simulink model "EvitarObstaculo"  (R2023a)
settings: Solver=FixedStepAuto  StartTime=0.0  StopTime=100  FixedStep=Ts  RelTol=1e-3
values from neighbouring files (symbols this model uses):
  obsx = 3    [RunTrayectorias.m]
  obsy = 2    [RunTrayectorias.m]
  Ts = 100e-3    (= 0.1)    [RunTrayectorias.m]
undefined symbols (not defined in the file or in its folder): DiscIntNeverNeededParam, refx, refy
libraries: fuzblock x1
settings Model: Creator=Edu  LastModifiedBy=Edu
settings DataIOCC: ReturnWorkspaceOutputs=off

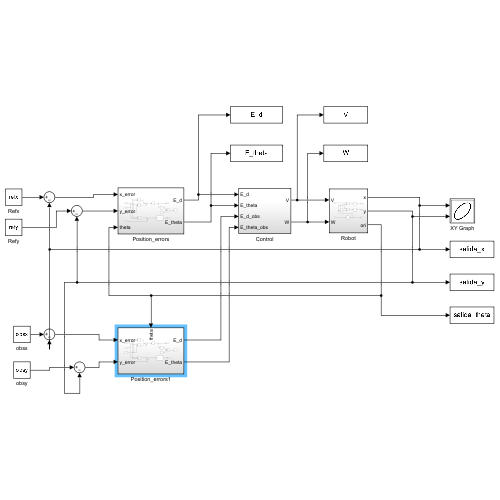
[thumbnail: Simulink's stored preview of the top-level diagram]
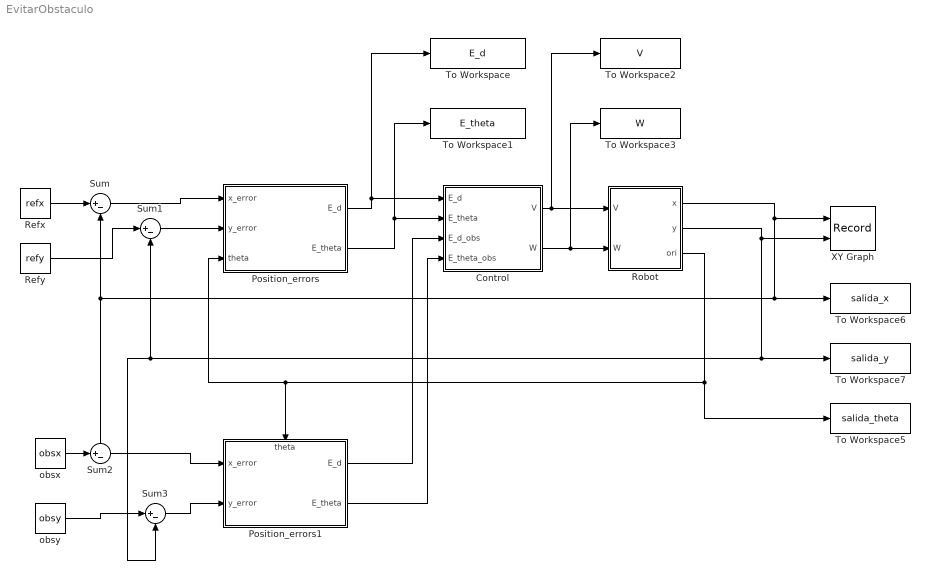
== system EvitarObstaculo ==
  Control : Subsystem
  Position_errors : Subsystem
  Position_errors1 : Subsystem
      settings: PortSchema="{\"entries\":[{\"content\":{\"sides\":[{\"content\":{\"connectorIds\":[\"In1\",\"In2\"]},\"type\":\"ConnectorPlacement.EquallySpacedRectSide\",\"uuid\":\"724a1adf-34fd-47e8-8329-3234fcffba95\"},{\"content\":{\"connectorIds\":[\"Out1\",\"Out2\"],\"side\":\"RIGHT\"},\"type\":\"ConnectorPlacement.EquallySpacedRectSide\",\"uuid\":\"8963bb18-06e6-4569-9caa-12a8dca62f16\"},{\"content\":{\"connectorIds\":[\"In3\"],\"side\":\"TOP\"},\"type\":\"ConnectorPlacement.EquallySpacedRectSide\",\"uuid\":\"b639e4b5-9e5a-472e-9105-86d06ea8a990\"}]},\"type\":\"ConnectorPlacement.EquallySpacedConnector\",\"uuid\":\"88dc6a9c-ca86-465e-ac65-937620f59bbe\"}],\"packageUris\":[\"http://schema.mathworks.com/mf0/Connector/R2020b\"],\"version\":\"1.0\"}"
  Refx : Constant  Value=refx
  Refy : Constant  Value=refy
  Robot : Subsystem
  Sum{,1..3} (4 alike) : Sum  Inputs=|+-
  To Workspace : ToWorkspace  VariableName=E_d  SaveFormat=Structure With Time  SampleTime=-1
  To Workspace1 : ToWorkspace  VariableName=E_theta  SaveFormat=Structure With Time  SampleTime=-1
  To Workspace2 : ToWorkspace  VariableName=V  SaveFormat=Structure With Time  SampleTime=-1
  To Workspace3 : ToWorkspace  VariableName=W  SaveFormat=Structure With Time  SampleTime=-1
  To Workspace5 : ToWorkspace  VariableName=salida_theta  SaveFormat=Structure With Time  SampleTime=-1
  To Workspace6 : ToWorkspace  VariableName=salida_x  SaveFormat=Structure With Time  SampleTime=-1
  To Workspace7 : ToWorkspace  VariableName=salida_y  SaveFormat=Structure With Time  SampleTime=-1
  XY Graph : Record  FileSettingsInternal="{\"entries\":[{\"content\":{\"excelSettings\":{\"content\":{},\"type\":\"Streamout.ExcelSettings\"}},\"type\":\"Streamout.FileSettingStorage\",\"uuid\":\"\"}],\"packageUris\":[\"http:\\/\\/schema.mathworks.com\\/mf0\\/streamout_blocks\\/R2020a\"],\"version\":\"1.0\"}"  Layout=[1 1]  SignalsInternal="{\"entries\":[{\"content\":{\"signals\":[{\"content\":{\"blockPath\":[],\"dimensions\":[1],\"domain\":\"\",\"lineColor\":\"#a2142f\",\"plots\":[1],\"port\":1,\"sid\":[\"\"],\"signalID\":3541,\"signalName\":\"Robot:1\"},\"type\":\"RecordBlkView.Signal\",\"uuid\":\"\"},{\"content\":{\"blockPath\":[],\"dimensions\":[1],\"domain\":\"\",\"lineColor\":\"#139fff\",\"plots\":[1],\"port\":2,\"sid\":[\"\"],\"signalID\":3545,\"signalName\":\"Robot:2\"},\"type\":\"RecordBlkView.Signal\",\"uuid\":\"\"}]},\"type\":\"RecordBlkView.InputSignals\",\"uuid\":\"\"}],\"packageUris\":[\"http:\\/\\/schema.mathworks.com\\/mf0\\/streamout_blocks\\/R2020a\"],\"version\":\"1.0\"}"  VisualizationBindings="{\"xyplotplugin\":{\"info\":[{\"series\":[{\"bindingParametersList\":[{\"parameter\":\"X-Axis\",\"signalID\":3541,\"signalName\":\"Robot:1\"},{\"parameter\":\"Y-Axis\",\"signalID\":3545,\"signalName\":\"Robot:2\"}],\"seriesID\":31515}],\"subplotID\":1}]}}"  CompatibilityTag=XY
  obsx : Constant  Value=obsx
  obsy : Constant  Value=obsy
  wires:
  Position_errors/2(E_theta) -> To Workspace1/1, Control/2(E_theta)
  Refy/1 -> Sum1/1
  Refx/1 -> Sum/1
  Control/1(V) -> To Workspace2/1, Robot/1(V)
  Position_errors/1(E_d) -> To Workspace/1, Control/1(E_d)
  Robot/2(y) -> To Workspace7/1, Sum3/2, Sum1/2, XY Graph/2
  Robot/3(ori) -> To Workspace5/1, Position_errors/3(theta), Position_errors1/3(theta)
  Control/2(W) -> To Workspace3/1, Robot/2(W)
  Sum/1 -> Position_errors/1(x_error)
  Sum1/1 -> Position_errors/2(y_error)
  Robot/1(x) -> Sum/2, Sum2/2, To Workspace6/1, XY Graph/1
  obsx/1 -> Sum2/1
  obsy/1 -> Sum3/1
  Sum2/1 -> Position_errors1/1(x_error)
  Sum3/1 -> Position_errors1/2(y_error)
  Position_errors1/2(E_theta) -> Control/4(E_theta_obs)
  Position_errors1/1(E_d) -> Control/3(E_d_obs)

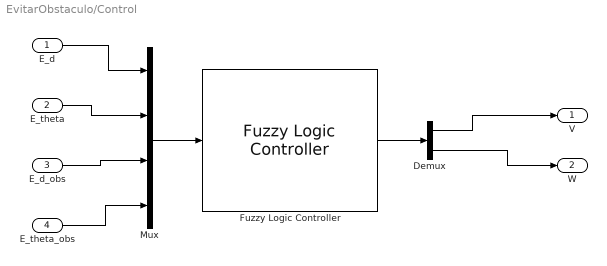
== system EvitarObstaculo/Control ==
  E_d : Inport
  E_theta : Inport  Port=2
  E_d_obs : Inport  Port=3
  E_theta_obs : Inport  Port=4
  Demux : Demux  Outputs=2
  Fuzzy Logic Controller : fuzblock/Fuzzy Logic  Controller  FIS='ControlBorroso2.fis'  OutputSampleNumber=101  DataType=double  FuzzifiedInputs=off  RuleFiringStrengths=off  RuleOutputs=off  AggregatedOutputs=off  SimulateUsing=Interpreted execution  OutOfRangeInputValueMessage=warning  NoRuleFiredMessage=warning  EmptyOutputFuzzySetMessage=warning
  Mux : Mux
  V : Outport  VectorParamsAs1DForOutWhenUnconnected=off
  W : Outport  Port=2  VectorParamsAs1DForOutWhenUnconnected=off
  wires:
  Mux/1 -> Fuzzy Logic Controller/1
  E_d/1 -> Mux/1
  E_theta/1 -> Mux/2
  Demux/1 -> V/1
  Demux/2 -> W/1
  Fuzzy Logic Controller/1 -> Demux/1
  E_d_obs/1 -> Mux/3
  E_theta_obs/1 -> Mux/4

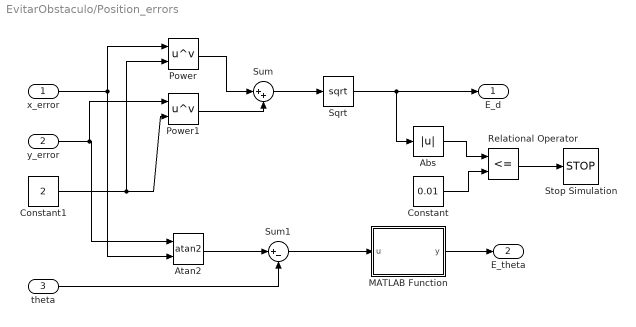
== system EvitarObstaculo/Position_errors ==
  x_error : Inport
  y_error : Inport  Port=2
  theta : Inport  Port=3
  Abs : Abs  SaturateOnIntegerOverflow=off
  Atan2 : Trigonometry  Operator=atan2
  Constant : Constant  Value=0.01
  Constant1 : Constant  Value=2
  MATLAB Function : MATLAB Function  TreatAsAtomicUnit=on
  Power : Math  Operator=pow
  Power1 : Math  Operator=pow
  Relational Operator : RelationalOperator  Operator=<=  OutDataTypeStr=boolean  RndMeth=Simplest  InputSameDT=off
  Sqrt : Sqrt
  Stop Simulation : Stop
  Sum : Sum  Inputs=|++
  Sum1 : Sum  Inputs=|+-
  E_d : Outport
  E_theta : Outport  Port=2
  wires:
  x_error/1 -> Atan2/2, Power/1
  y_error/1 -> Atan2/1, Power1/1
  Sum/1 -> Sqrt/1
  Sqrt/1 -> Abs/1, E_d/1
  Atan2/1 -> Sum1/1
  theta/1 -> Sum1/2
  Sum1/1 -> MATLAB Function/1(u)
  Relational Operator/1 -> Stop Simulation/1
  Abs/1 -> Relational Operator/1
  Constant/1 -> Relational Operator/2
  MATLAB Function/1(y) -> E_theta/1
  Constant1/1 -> Power/2, Power1/2
  Power1/1 -> Sum/2
  Power/1 -> Sum/1

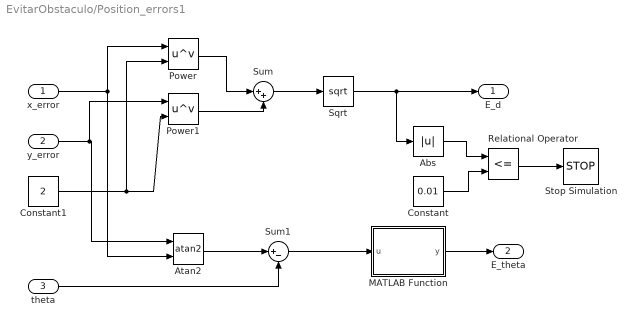
== system EvitarObstaculo/Position_errors1 ==
  x_error : Inport
  y_error : Inport  Port=2
  theta : Inport  Port=3
  Abs : Abs  SaturateOnIntegerOverflow=off
  Atan2 : Trigonometry  Operator=atan2
  Constant : Constant  Value=0.01
  Constant1 : Constant  Value=2
  MATLAB Function : MATLAB Function  TreatAsAtomicUnit=on
  Power : Math  Operator=pow
  Power1 : Math  Operator=pow
  Relational Operator : RelationalOperator  Operator=<=  OutDataTypeStr=boolean  RndMeth=Simplest  InputSameDT=off
  Sqrt : Sqrt
  Stop Simulation : Stop
  Sum : Sum  Inputs=|++
  Sum1 : Sum  Inputs=|+-
  E_d : Outport
  E_theta : Outport  Port=2
  wires:
  x_error/1 -> Atan2/2, Power/1
  y_error/1 -> Atan2/1, Power1/1
  Sum/1 -> Sqrt/1
  Sqrt/1 -> Abs/1, E_d/1
  Atan2/1 -> Sum1/1
  theta/1 -> Sum1/2
  Sum1/1 -> MATLAB Function/1(u)
  Relational Operator/1 -> Stop Simulation/1
  Abs/1 -> Relational Operator/1
  Constant/1 -> Relational Operator/2
  MATLAB Function/1(y) -> E_theta/1
  Constant1/1 -> Power/2, Power1/2
  Power1/1 -> Sum/2
  Power/1 -> Sum/1

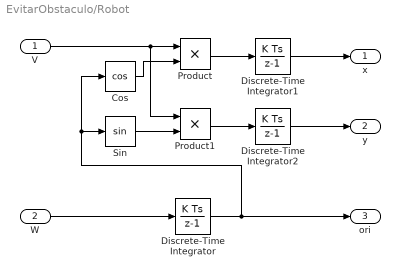
== system EvitarObstaculo/Robot ==
  V : Inport
  W : Inport  Port=2
  Cos : Trigonometry  Operator=cos
  Discrete-Time Integrator : DiscreteIntegrator  SampleTime=Ts  ICPrevOutput=DiscIntNeverNeededParam  ICPrevScaledInput=DiscIntNeverNeededParam
  Discrete-Time Integrator1 : DiscreteIntegrator  SampleTime=Ts  ICPrevOutput=DiscIntNeverNeededParam  ICPrevScaledInput=DiscIntNeverNeededParam
  Discrete-Time Integrator2 : DiscreteIntegrator  SampleTime=Ts  ICPrevOutput=DiscIntNeverNeededParam  ICPrevScaledInput=DiscIntNeverNeededParam
  Product : Product
  Product1 : Product
  Sin : Trigonometry
  x : Outport
  y : Outport  Port=2
  ori : Outport  Port=3
  wires:
  Discrete-Time Integrator/1 -> ori/1, Sin/1, Cos/1
  Discrete-Time Integrator1/1 -> x/1
  Cos/1 -> Product/2
  V/1 -> Product1/1, Product/1
  Sin/1 -> Product1/2
  Discrete-Time Integrator2/1 -> y/1
  W/1 -> Discrete-Time Integrator/1
  Product1/1 -> Discrete-Time Integrator2/1
  Product/1 -> Discrete-Time Integrator1/1

== matlab function EvitarObstaculo/Position_errors/MATLAB Function ==
  data: u input; y output
%function y = tranformar(u)
%if(u>3*pi) 
%y=u-4*pi;
%elseif (u>pi)
%y=u-2*pi;
%elseif(u<-3*pi) 
%y=u+4*pi ;
%elseif(u<-pi)
%y=u+2*pi ;
%else 
%y=u;
%end

function y = transformar(u)

if (u > pi)
    y = u - 2*pi;
elseif (u < -pi)
    y = u + 2*pi;
else
    y = u;
end

== matlab function EvitarObstaculo/Position_errors1/MATLAB Function ==
  data: u input; y output
%function y = tranformar(u)
%if(u>3*pi) 
%y=u-4*pi;
%elseif (u>pi)
%y=u-2*pi;
%elseif(u<-3*pi) 
%y=u+4*pi ;
%elseif(u<-pi)
%y=u+2*pi ;
%else 
%y=u;
%end 

function y = transformar(u)

if (u > pi)
    y = u - 2*pi;
elseif (u < -pi)
    y = u + 2*pi;
else
    y = u;
end
